simulink model "clik_z_inverse"  (R2022b)
settings: Solver=ode1  StartTime=0.0  StopTime=4  FixedStep=0.001  RelTol=1e-3
undefined symbols (not defined in the file or in its folder): DiscIntNeverNeededParam, q0, Tc
settings Model: Creator=Xp  LastModifiedBy=DELL
settings SolverCC: AlgebraicLoopSolver=TrustRegion
settings DataIOCC: LimitDataPoints=on  SaveFormat=Array  SignalLoggingSaveFormat=ModelDataLogs  ReturnWorkspaceOutputs=off
settings OptimizationCC: ExpressionDepthLimit=2147483647  InitFltsAndDblsToZero=on  LifeSpan=inf
settings DebuggingCC: SaveWithParameterizedLinksMsg=none  UnderspecifiedInitializationDetection=Classic  MergeDetectMultiDrivingBlocksExec=none  SolverPrmCheckMsg=warning  MultiTaskDSMMsg=warning  MultiTaskCondExecSysMsg=none  FcnCallInpInsideContextMsg=warning  UnconnectedInputMsg=warning  UnconnectedOutputMsg=warning  UnconnectedLineMsg=warning  StateNameClashWarn=warning  SFUnexpectedBacktrackingDiag=warning  SFNoUnconditionalDefaultTransitionDiag=warning  SFExecutionAtInitializationDiag=none  SFMachineParentedDataDiag=warning  ArithmeticOperatorsInVariantConditions=warning
settings HardwareCC: ProdBitPerPointer=32  ProdBitPerSizeT=32  ProdBitPerPtrDiffT=32  ProdLargestAtomicFloat=None  ProdIntDivRoundTo=Undefined  ProdEndianess=Unspecified  ProdWordSize=32  ProdHWDeviceType=32-bit Generic
settings ModelReferenceCC: EnableRefExpFcnMdlSchedulingChecks=on  PropagateSignalLabelsOutOfModel=off
settings SFSimCC: CustomCodeUndefinedFunction=UseInterfaceOnly
settings RTWCC: DLArmComputeVersion=19.05
settings CodeAppCC: StateflowObjectComments=on
settings GRTTargetCC: TargetLangStandard=C89/C90 (ANSI)  CombineOutputUpdateFcns=off  GRTInterface=on
settings ConfigComp: CovMetricSettings=dw  CovSaveCumulativeToWorkspaceVar=on  CovSaveSingleToWorkspaceVar=on

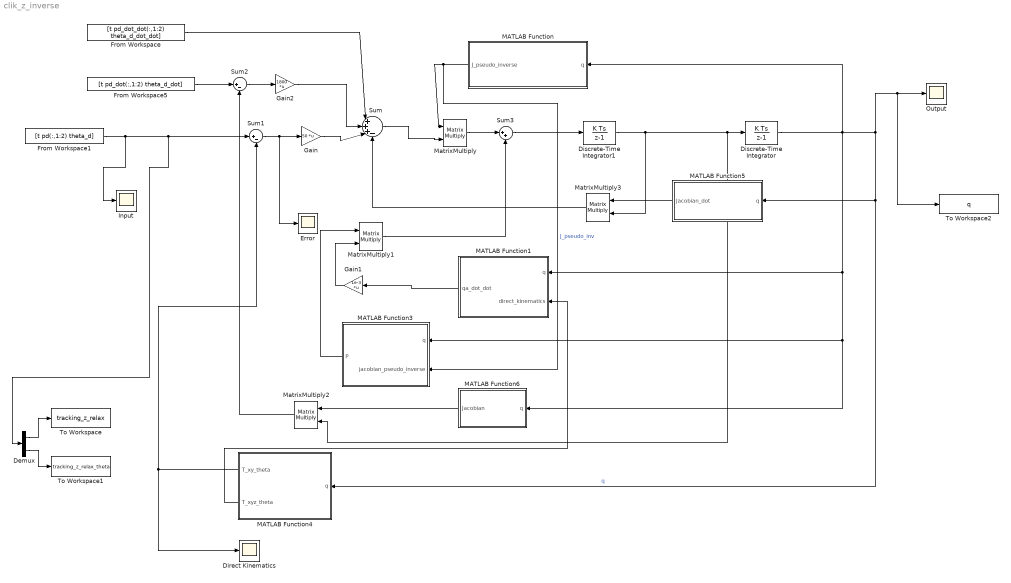
== system clik_z_inverse ==
  Demux : Demux  Outputs=2
  Direct Kinematics : Scope
  Discrete-Time Integrator : DiscreteIntegrator  InitialCondition=q0  SampleTime=Tc  LimitOutput=on  UpperSaturationLimit=[pi/2;pi/4;1;2*pi]  LowerSaturationLimit=[-pi/2;-pi/2;0.25;-2*pi]  ICPrevOutput=DiscIntNeverNeededParam  ICPrevScaledInput=DiscIntNeverNeededParam
  Discrete-Time Integrator1 : DiscreteIntegrator  SampleTime=Tc  UpperSaturationLimit=[pi/2;pi/4;1;2*pi]  LowerSaturationLimit=[-pi/2;-pi/2;0.25;-2*pi]  ICPrevOutput=DiscIntNeverNeededParam  ICPrevScaledInput=DiscIntNeverNeededParam
  Error : Scope
  From Workspace : FromWorkspace  VariableName=[t pd_dot_dot(:,1:2) theta_d_dot_dot]  SampleTime=Tc
  From Workspace1 : FromWorkspace  VariableName=[t pd(:,1:2) theta_d]  SampleTime=Tc
  From Workspace5 : FromWorkspace  VariableName=[t pd_dot(:,1:2) theta_d_dot]  SampleTime=Tc
  Gain : Gain  Gain=50  Multiplication=Matrix(K*u)
  Gain1 : Gain  Gain=1e-3  Multiplication=Matrix(K*u)
  Gain2 : Gain  Gain=1800  Multiplication=Matrix(K*u)
  Input : Scope
  MATLAB Function : MATLAB Function  TreatAsAtomicUnit=on
  MATLAB Function1 : MATLAB Function  TreatAsAtomicUnit=on
  MATLAB Function3 : MATLAB Function  TreatAsAtomicUnit=on
  MATLAB Function4 : MATLAB Function  TreatAsAtomicUnit=on
  MATLAB Function5 : MATLAB Function  TreatAsAtomicUnit=on
  MATLAB Function6 : MATLAB Function  TreatAsAtomicUnit=on
  MatrixMultiply{,1..3} (4 alike) : Product  Multiplication=Matrix(*)
  Output : Scope
  Sum : Sum  Inputs=|+++-
  Sum1 : Sum  Inputs=|+-
  Sum2 : Sum  Inputs=|+-
  Sum3 : Sum  Inputs=|++
  To Workspace : ToWorkspace  VariableName=tracking_z_relax  SampleTime=Tc
  To Workspace1 : ToWorkspace  VariableName=tracking_z_relax_theta  SampleTime=Tc
  To Workspace2 : ToWorkspace  VariableName=q  SampleTime=Tc
  wires:
  Gain2/1 -> Sum/2
  Discrete-Time Integrator1/1 -> MatrixMultiply3/2, MatrixMultiply2/2, Discrete-Time Integrator/1
  Sum2/1 -> Gain2/1
  MatrixMultiply3/1 -> Sum/4
  MATLAB Function6/1(Jacobian) -> MatrixMultiply2/1
  From Workspace5/1 -> Sum2/1
  From Workspace/1 -> Sum/1
  MatrixMultiply2/1 -> Sum2/2
  MATLAB Function5/1(Jacobian_dot) -> MatrixMultiply3/1
  Gain/1 -> Sum/3
  Sum1/1 -> Error/1, Gain/1
  Discrete-Time Integrator/1 -> MATLAB Function1/1(q), MATLAB Function6/1(q), MATLAB Function3/1(q), MATLAB Function/1(q), MATLAB Function5/1(q), MATLAB Function4/1(q), To Workspace2/1, Output/1  "q"
  MATLAB Function/1(J_pseudo_inverse) -> MATLAB Function3/2(jacobian_pseudo_inverse), MatrixMultiply/1  "J_pseudo_inv"
  MatrixMultiply/1 -> Sum3/1
  Sum3/1 -> Discrete-Time Integrator1/1
  MATLAB Function3/1(P) -> MatrixMultiply1/1
  MatrixMultiply1/1 -> Sum3/2
  MATLAB Function4/1(T_xy_theta) -> Sum1/2, Direct Kinematics/1
  MATLAB Function4/2(T_xyz_theta) -> MATLAB Function1/2(direct_kinematics)
  Gain1/1 -> MatrixMultiply1/2
  Sum/1 -> MatrixMultiply/2
  From Workspace1/1 -> Demux/1, Sum1/1, Input/1
  MATLAB Function1/1(qa_dot_dot) -> Gain1/1
  Demux/1 -> To Workspace/1
  Demux/2 -> To Workspace1/1

== matlab function clik_z_inverse/MATLAB Function1 ==
  data: q input; qa_dot_dot output; direct_kinematics input
function qa_dot_dot = qa_dot_dot_function_call(q, direct_kinematics)

% Center co-ordinates of the obstacle(Sphere in this case)
% These co-ordinates are after adding the radius of the sphere to them which
% is 0.2m since the end effector of the manipulator has to be at the
% maximum possible distance from the outer surface of the sphere
p_obstacle = [0.6; -0.5; 0.7];

% Initialzing w
w = zeros(4,1);

for i = 1:4

    norm_result = norm(direct_kinematics - p_obstacle);

    w(i) = norm_result;
    
end

% Finding first order differential qa_dot
qa_dot = gradient(w,q);

% Finding second order differential qa_dot_dot
qa_dot_dot = gradient(qa_dot,q);

== matlab function clik_z_inverse/MATLAB Function ==
  data: q input; J_pseudo_inverse output
function J_pseudo_inverse = jacobian_pseudo_inverse(q)

% Calling the jacobian function from the jacobian matlab file
J = jacobian_z_relax(q);

% Calculating tranpose of jacobian matrix
J_transpose = transpose(J);

JJ_transpose = J * J_transpose;

JJ_transpose_inverse = inv(JJ_transpose);

% Finally calculating pseudo-inverse of jacobian matrix
J_pseudo_inverse = J_transpose * JJ_transpose_inverse;

== matlab function clik_z_inverse/MATLAB Function3 ==
  data: q input; P output; jacobian_pseudo_inverse input
function P = p_matrix(q, jacobian_pseudo_inverse)

% Caling the jacobian_z_relax function to get the jacobian matrix
jacobian = jacobian_z_relax(q);


product = jacobian_pseudo_inverse * jacobian;

% Finding the P matrix
P = eye(4,4) - product;

== matlab function clik_z_inverse/MATLAB Function4 ==
  data: q input; T_xy_theta output; T_xyz_theta output
function [T_xy_theta, T_xyz_theta] = direct_kin(q)

% Defining link length values
a1 = 0.5;
a2 = 0.5;
d0 = 1;

% Assigning individual joint values to the corresponding rows of the
% q(angle) being taken as input
q1=q(1);
q2=q(2);
d3=q(3);
q4=q(4);

% Obtained Rotation and translation direct kinematics matrix for scara manipulator
R=[cos(q1+q2+q4),sin(q1+q2+q4),0;sin(q1+q2+q4),-cos(q1+q2+q4),0;0,0,-1;0 0 0];
T_xy_theta=[a1*cos(q1)+a2*cos(q1+q2);a1*sin(q1)+a2*sin(q1+q2);q1+q2+q4]; % Here we are passing only X, Y and theta since Z is relaxed

T_xyz_theta = [a1*cos(q1)+a2*cos(q1+q2);a1*sin(q1)+a2*sin(q1+q2);-d3+d0]; % Passing all the X, Y, Z and theta for subtracing from the obstacle co-ordinates

== matlab function clik_z_inverse/MATLAB Function5 ==
  data: q input; Jacobian_dot output
function Jacobian_dot = jacobian_dot(q)

% Caling the jacobian_dot function to find the first order differential of jacobian matrix
Jacobian_dot = jacobian_dot(q);

== matlab function clik_z_inverse/MATLAB Function6 ==
  data: q input; Jacobian output
function Jacobian = jacobian_z_relax(q)

% Caling the jacobian_z_relax function to get the jacobian matrix
Jacobian = jacobian_z_relax(q);
